simulink model "RCAM_Simulation"  (R2021b)
settings: Solver=VariableStepAuto  StartTime=0.0  StopTime=TF  RelTol=1e-3
values from neighbouring files (symbols this model uses):
  a = 6378137.0    (= 6378137)    [Setup_RCAM_Joystick_Flightgear.m]
  e = 0.08181919084622    (= 0.0818191908462)    [Setup_RCAM_Joystick_Flightgear.m]
  h = 700    [Setup_RCAM_Joystick_Flightgear.m]
  lat = 47.608013*pi/180    (= 0.830916577182)    [Setup_RCAM_Joystick_Flightgear.m]
  long = -122.335167*pi/180    (= -2.13515145513)    [Setup_RCAM_Joystick_Flightgear.m]
  u0 = uSolve    [Setup_RCAM_Joystick_Flightgear.m]
  x0 = xSolve    [Setup_RCAM_Joystick_Flightgear.m]
undefined symbols (not defined in the file or in its folder): Calculate_Cvb, RCAM_model_D
libraries: aerolibfltsims x2, aerolibanimutils x2
settings Model: Creator=Aidan  LastModifiedBy=Aidan

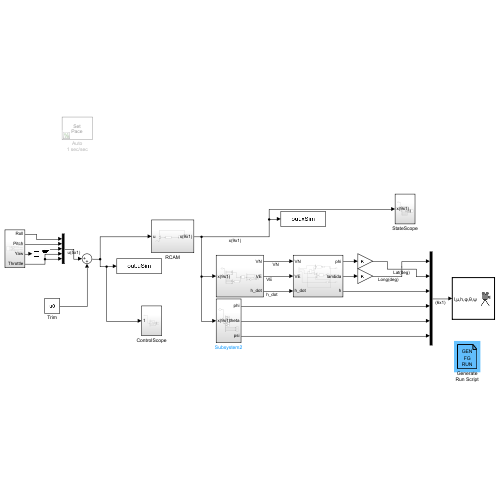
[thumbnail: Simulink's stored preview of the top-level diagram]
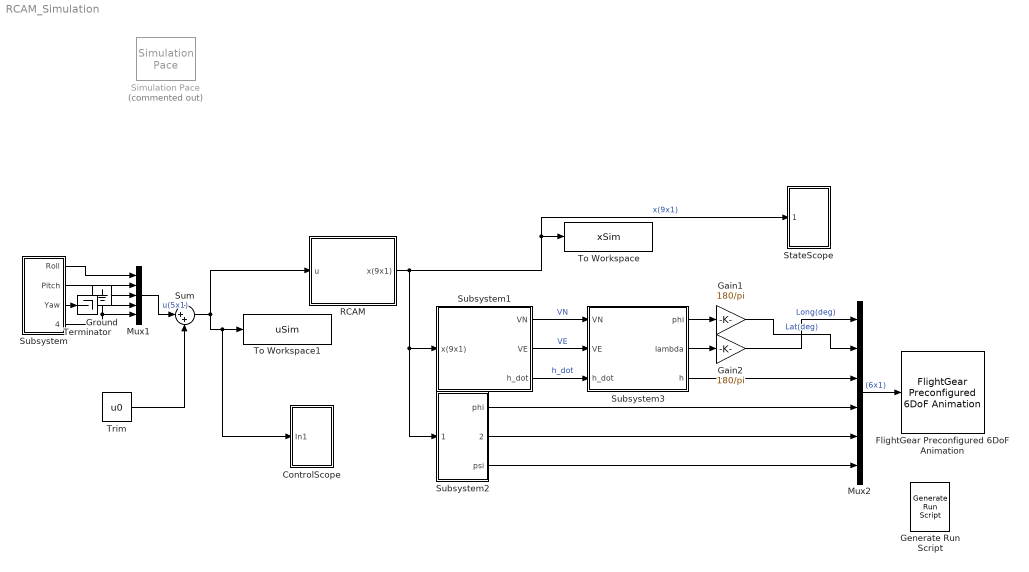
== system RCAM_Simulation ==
  ControlScope : Subsystem
  FlightGear Preconfigured 6DoF Animation : aerolibfltsims/FlightGear Preconfigured 6DoF Animation  xFlightGearVersion=v2019.1  DestinationIpAddress=127.0.0.1  DestinationPort=5502  SampleTime=1/30  packetVersion=24
  Gain1 : Gain  Gain=180/pi
  Gain2 : Gain  Gain=180/pi
  Generate Run Script : aerolibfltsims/Generate Run Script  Architecture=Win64  dataFlow=Send  GeometryModelName=c172p  AirportId=KSFO  RunwayId=10L  InitialAltitude=7224  InitialHeading=113  OffsetDistance=4.72  OffsetAzimuth=0  InstallScenery=off  DisableShaders=on  OriginAddress=127.0.0.1  DestinationPort=5502  OriginPort=5505  LocalAddress=127.0.0.1  OutputFileName=runfg.bat  FlightGearBaseDirectory=C:\Program Files\FlightGear 2020.3
  Ground : Ground
  Mux1 : Mux  Inputs=5
  Mux2 : Mux  Inputs=6
  RCAM : Subsystem
  Simulation Pace : aerolibanimutils/Simulation Pace  Commented=on  SimulationPace=1  SleepMode=Auto  OutputPaceError=off  SampleTime=1/30
  StateScope : Subsystem
  Subsystem : Subsystem
  Subsystem1 : Subsystem
  Subsystem2 : Subsystem
  Subsystem3 : Subsystem
  Sum : Sum  Inputs=|++
  Terminator : Terminator
  To Workspace : ToWorkspace  VariableName=xSim  SaveFormat=Structure  SampleTime=-1
      settings: Save2DSignal=2-D array (concatenate along first dimension)
  To Workspace1 : ToWorkspace  VariableName=uSim  SaveFormat=Structure  SampleTime=-1
      settings: Save2DSignal=2-D array (concatenate along first dimension)
  Trim : Constant  Value=u0
  wires:
  Sum/1 -> RCAM/1(u), ControlScope/1(In1), To Workspace1/1
  Subsystem/1(Roll) -> Mux1/1
  Subsystem/2(Pitch) -> Mux1/2
  Subsystem/4(Throttle) -> Mux1/5, Mux1/4
  Trim/1 -> Sum/2
  Ground/1 -> Mux1/3
  Mux1/1 -> Sum/1  "u(5x1)"
  RCAM/1(x(9x1)) -> Subsystem2/1(x(9x1)), Subsystem1/1(x(9x1)), To Workspace/1, StateScope/1(x(9x1))  "x(9x1)"
  Subsystem1/1(VN) -> Subsystem3/1(VN)  "VN"
  Subsystem1/2(VE) -> Subsystem3/2(VE)  "VE"
  Subsystem1/3(h_dot) -> Subsystem3/3(h_dot)  "h_dot"
  Subsystem3/3(h) -> Mux2/3
  Subsystem2/1(phi) -> Mux2/4
  Subsystem2/2(theta) -> Mux2/5
  Subsystem2/3(psi) -> Mux2/6
  Mux2/1 -> FlightGear Preconfigured 6DoF Animation/1  "(6x1)"
  Subsystem3/2(lambda) -> Gain2/1
  Subsystem3/1(phi) -> Gain1/1
  Gain2/1 -> Mux2/1  "Long(deg)"
  Gain1/1 -> Mux2/2  "Lat(deg)"
  Subsystem/3(Yaw) -> Terminator/1

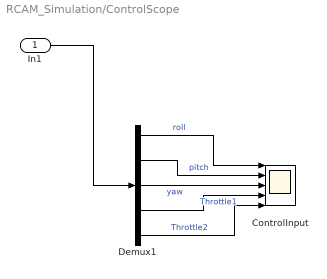
== system RCAM_Simulation/ControlScope ==
  In1 : Inport
  ControlInput : Scope  NumInputPorts=5
  Demux1 : Demux  Outputs=5
  wires:
  Demux1/3 -> ControlInput/3  "yaw"
  Demux1/5 -> ControlInput/5  "Throttle2"
  Demux1/4 -> ControlInput/4  "Throttle1"
  In1/1 -> Demux1/1
  Demux1/1 -> ControlInput/1  "roll"
  Demux1/2 -> ControlInput/2  "pitch"

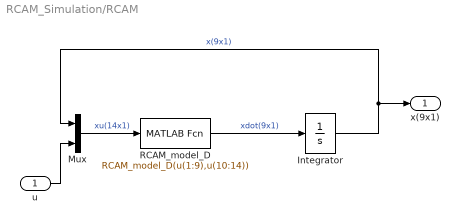
== system RCAM_Simulation/RCAM ==
  u : Inport
  Integrator : Integrator  InitialCondition=x0
  Mux : Mux  Inputs=2
  RCAM_model_D : MATLABFcn  MATLABFcn=RCAM_model_D(u(1:9),u(10:14))
  x(9x1) : Outport
  wires:
  Integrator/1 -> x(9x1)/1, Mux/1  "x(9x1)"
  RCAM_model_D/1 -> Integrator/1  "xdot(9x1)"
  Mux/1 -> RCAM_model_D/1  "xu(14x1)"
  u/1 -> Mux/2

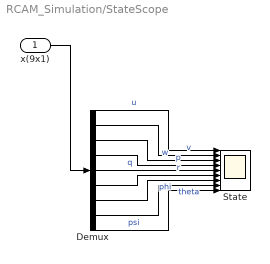
== system RCAM_Simulation/StateScope ==
  x(9x1) : Inport
  Demux : Demux  Outputs=9
  State : Scope  NumInputPorts=9
  wires:
  Demux/5 -> State/5  "q"
  Demux/8 -> State/8  "theta"
  Demux/3 -> State/3  "w"
  Demux/4 -> State/4  "p"
  Demux/7 -> State/7  "phi"
  Demux/6 -> State/6  "r"
  Demux/9 -> State/9  "psi"
  Demux/1 -> State/1  "u"
  x(9x1)/1 -> Demux/1
  Demux/2 -> State/2  "v"

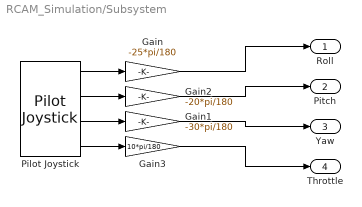
== system RCAM_Simulation/Subsystem ==
  Gain : Gain  Gain=-25*pi/180
  Gain1 : Gain  Gain=-30*pi/180
  Gain2 : Gain  Gain=-20*pi/180
  Gain3 : Gain  Gain=10*pi/180
  Pilot Joystick : aerolibanimutils/Pilot Joystick  JoystickID=Joystick1  OutputConfiguration=FourAxis  SampleTime=1/30
  Roll : Outport
  Pitch : Outport  Port=2
  Yaw : Outport  Port=3
  Throttle : Outport  Port=4
  wires:
  Pilot Joystick/2 -> Gain2/1
  Pilot Joystick/3 -> Gain1/1
  Gain2/1 -> Pitch/1
  Pilot Joystick/1 -> Gain/1
  Gain/1 -> Roll/1
  Pilot Joystick/4 -> Gain3/1
  Gain3/1 -> Throttle/1
  Gain1/1 -> Yaw/1

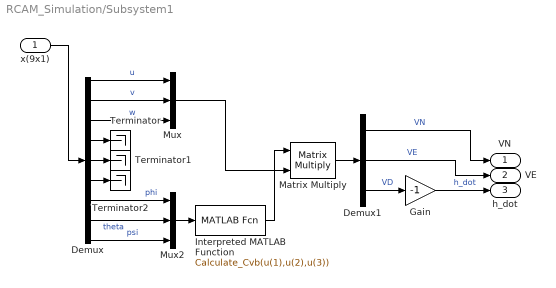
== system RCAM_Simulation/Subsystem1 ==
  x(9x1) : Inport
  Demux : Demux  Outputs=9
  Demux1 : Demux  Outputs=3
  Gain : Gain  Gain=-1
  Interpreted MATLAB Function : MATLABFcn  MATLABFcn=Calculate_Cvb(u(1),u(2),u(3))  Output1D=off
  Matrix Multiply : Product  Multiplication=Matrix(*)
  Mux : Mux  Inputs=3
  Mux2 : Mux  Inputs=3
  Terminator : Terminator
  Terminator1 : Terminator
  Terminator2 : Terminator
  VN : Outport
  VE : Outport  Port=2
  h_dot : Outport  Port=3
  wires:
  Demux1/3 -> Gain/1  "VD"
  Demux/4 -> Terminator/1
  Demux/1 -> Mux/1  "u"
  Demux/5 -> Terminator1/1
  Demux/3 -> Mux/3  "w"
  Demux/2 -> Mux/2  "v"
  Interpreted MATLAB Function/1 -> Matrix Multiply/1
  Demux/9 -> Mux2/3  "psi"
  Mux2/1 -> Interpreted MATLAB Function/1
  Demux/8 -> Mux2/2  "theta"
  Demux/7 -> Mux2/1  "phi"
  Matrix Multiply/1 -> Demux1/1
  Mux/1 -> Matrix Multiply/2
  x(9x1)/1 -> Demux/1
  Demux/6 -> Terminator2/1
  Demux1/1 -> VN/1  "VN"
  Gain/1 -> h_dot/1  "h_dot"
  Demux1/2 -> VE/1  "VE"

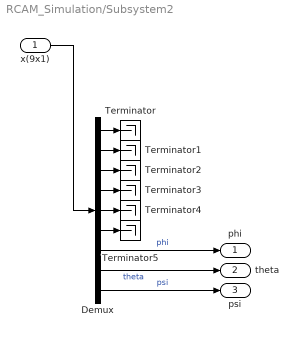
== system RCAM_Simulation/Subsystem2 ==
  x(9x1) : Inport
  Demux : Demux  Outputs=9
  Terminator{,1..5} (6 alike) : Terminator
  phi : Outport
  theta : Outport  Port=2
  psi : Outport  Port=3
  wires:
  Demux/2 -> Terminator1/1
  Demux/3 -> Terminator2/1
  Demux/1 -> Terminator/1
  Demux/6 -> Terminator5/1
  Demux/5 -> Terminator4/1
  x(9x1)/1 -> Demux/1
  Demux/9 -> psi/1  "psi"
  Demux/4 -> Terminator3/1
  Demux/7 -> phi/1  "phi"
  Demux/8 -> theta/1  "theta"

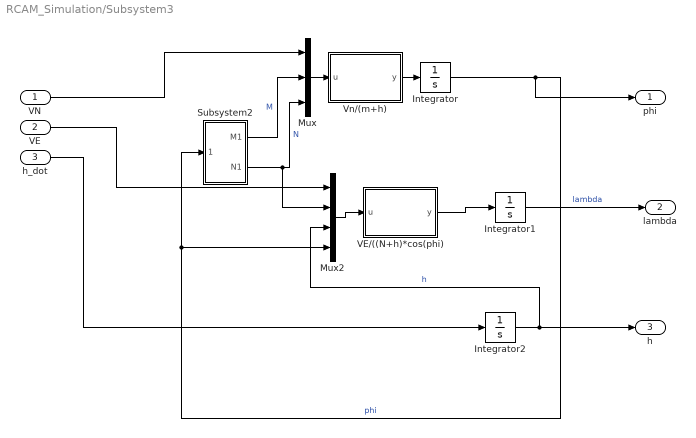
== system RCAM_Simulation/Subsystem3 ==
  VN : Inport
  VE : Inport  Port=2
  h_dot : Inport  Port=3
  Integrator : Integrator  InitialCondition=lat
  Integrator1 : Integrator  InitialCondition=long
  Integrator2 : Integrator  InitialCondition=h
  Mux : Mux  Inputs=3
  Mux2 : Mux
  Subsystem2 : Subsystem
  VE/((N+h)*cos(phi) : MATLAB Function  TreatAsAtomicUnit=on
  Vn/(m+h) : MATLAB Function  TreatAsAtomicUnit=on
  phi : Outport
  lambda : Outport  Port=2
  h : Outport  Port=3
  wires:
  Subsystem2/1(M1) -> Mux/2  "M"
  Subsystem2/2(N1) -> Mux2/2, Mux/3  "N"
  Integrator/1 -> phi/1, Subsystem2/1(phi), Mux2/4  "phi"
  Mux2/1 -> VE/((N+h)*cos(phi)/1(u)
  h_dot/1 -> Integrator2/1
  Integrator2/1 -> h/1, Mux2/3  "h"
  Vn/(m+h)/1(y) -> Integrator/1
  Mux/1 -> Vn/(m+h)/1(u)
  VE/((N+h)*cos(phi)/1(y) -> Integrator1/1
  Integrator1/1 -> lambda/1  "lambda"
  VN/1 -> Mux/1
  VE/1 -> Mux2/1

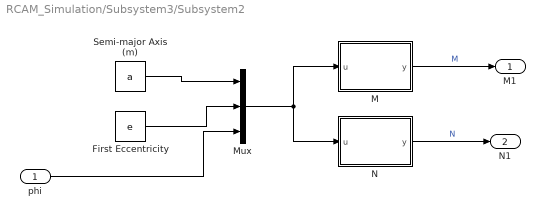
== system RCAM_Simulation/Subsystem3/Subsystem2 ==
  phi : Inport
  First Eccentricity : Constant  Value=e
  M : MATLAB Function  TreatAsAtomicUnit=on
  Mux : Mux  Inputs=3
  N : MATLAB Function  TreatAsAtomicUnit=on
  Semi-major Axis (m) : Constant  Value=a
  M1 : Outport
  N1 : Outport  Port=2
  wires:
  Mux/1 -> M/1(u), N/1(u)
  Semi-major Axis (m)/1 -> Mux/1
  phi/1 -> Mux/3
  First Eccentricity/1 -> Mux/2
  M/1(y) -> M1/1  "M"
  N/1(y) -> N1/1  "N"

== matlab function RCAM_Simulation/Subsystem3/Subsystem2/M ==
  data: u input; y output
function y = fcn(u)
    
y = u(1)*(1-(u(2)^2))/(1-(u(2)^2)*sin(u(3))^(2))^(3/2);

== matlab function RCAM_Simulation/Subsystem3/Vn//(m+h) ==
  data: u input; y output
function y = fcn(u)

y = u(1)/(u(2)+u(3));

== matlab function RCAM_Simulation/Subsystem3/VE//((N+h)*cos(phi) ==
  data: u input; y output
function y = fcn(u)

y = u(1)/((u(2)+u(3))*cos(u(4)));

== matlab function RCAM_Simulation/Subsystem3/Subsystem2/N ==
  data: u input; y output
function y = fcn(u)
    
y = u(1)/(1-u(2)^2*sin(u(3))^2)^(1/2);
